simulink model "Lab3"  (Simulink 7.1)
settings: Solver=ode45  SolverMode=SingleTasking  StartTime=0.0  StopTime=10.0  RelTol=1e-3  AbsTol=1e-6
settings Model: Creator=vise  LastModifiedBy=vise  ExtModeTrigMode=oneshot  ExtModeArmWhenConnect=off
settings DataIOCC: LimitDataPoints=off
settings OptimizationCC: BlockReduction=off  BooleanDataType=off
settings DebuggingCC: SaveWithParameterizedLinksMsg=none  SignalResolutionControl=TryResolveAllWithWarning  SolverPrmCheckMsg=none  MultiTaskDSMMsg=warning  MultiTaskCondExecSysMsg=none  StrictBusMsg=None
settings HardwareCC: TargetUnknown=on
settings RTWCC: TemplateMakefile=grt_unix.tmf  IncludeERTFirstTime=on

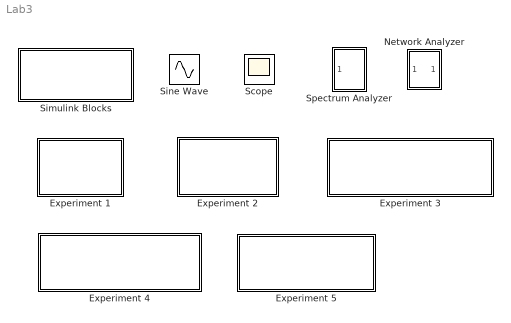
== system Lab3 ==
  Experiment 1 : Subsystem
      settings: OpenFcn=lab3Synth
      mask Type: Waveform Synthesizer
      mask Display: disp('Synthesizer')
  Experiment 2 : Subsystem
      settings: OpenFcn=lab3Mod
      mask Type: Modulator
      mask Display: disp('Modulator')
  Experiment 3 : Subsystem  Orientation=left
      settings: OpenFcn=lab3CTSys1
      mask Type: CT System Analysis/Network Analyzer
      mask Display: disp('CT System Analysis using\n a Network Analyzer')
  Experiment 4 : Subsystem
      settings: OpenFcn=lab3CTSys2
      mask Type: CT System Analysis/Unit Step
      mask Display: disp('CT System Analysis using\n a Unit Step')
  Experiment 5 : Subsystem
      settings: OpenFcn=lab3DTSys
      mask Type: DT System Analysis
      mask Display: disp('DT System Analysis')
  Network Analyzer : Subsystem  Orientation=left  mask(Network Analyzer){@1=256, @2=0.1}
      mask prompts: @1 "Number of sample points:"; @2 "Sampling period (sec):"
      mask init:
      | max_freq=0.9*pi/@2;N=@1;T_s=@2;const=2*pi/(@1*@2);window1=0.5*@1*@2;window2=@1*@2;
      mask Help: Estimates frequency response of system using chirp input. Used for EE438. See Prof. Bouman.
      mask Display: plot(0,0,100,100,[11,93,93,11,11],[90,90,40,40,90],[80,60,40,20],[50,79,50,80])
  Scope : Scope
      settings: TickLabels=on  DataFormat=Array
  Simulink Blocks : Subsystem
      settings: OpenFcn=simulink
      mask Type: Waveform Synthesizer
      mask Display: disp('Full Block Library')
  Sine Wave : Sin  SampleTime=0
  Spectrum Analyzer : Subsystem  mask(Spectrum analyzer.){@1=2048, @2=0.02, @3=10}
      mask prompts: @1 "Number of sample points:"; @2 "Sampling period (sec):"; @3 "Plotting Period (sec):"
      mask init:
      | N=@1; T_s=@2;plot_period=@3;
      mask Help: EE438 Lab utility; See Prof. Bouman.
      mask Display: plot(0,0,100,100,[14,91,91,14,14],[86,86,40,40,86],[85,82,80,79,75,67,63,60,57,53,41,36,33,27,24],[49,50,53,50,49,51,54,66,54,50,50,52,81,51,49])

== system Lab3/Experiment 1 ==

== system Lab3/Experiment 2 ==

== system Lab3/Experiment 3 ==

== system Lab3/Experiment 4 ==

== system Lab3/Experiment 5 ==

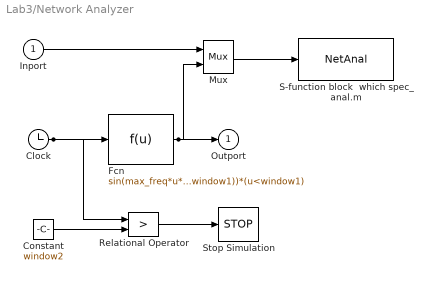
== system Lab3/Network Analyzer ==
  Inport : Inport
  Clock : Clock
      settings: Decimation=10
  Constant : Constant  Value=window2
  Fcn : Fcn  Expr=sin(max_freq*u*u/(2*window1))*(0.54+0.46*cos(pi*u/window1))*(u<window1)
  Mux : Mux  Inputs=2
  Relational Operator : RelationalOperator  Operator=>  InputSameDT=on
  S-function block  which spec_anal.m : S-Function  FunctionName=NetAnal  Parameters=N,T_s  EnableBusSupport=off
  Stop Simulation : Stop
  Outport : Outport  InitialOutput=0
  wires:
  Inport/1 -> Mux/1
  Fcn/1 -> Mux/2, Outport/1
  Mux/1 -> S-function block  which spec_anal.m/1
  Clock/1 -> Fcn/1, Relational Operator/1
  Constant/1 -> Relational Operator/2
  Relational Operator/1 -> Stop Simulation/1

== system Lab3/Simulink Blocks ==

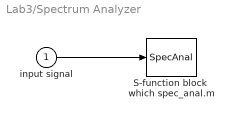
== system Lab3/Spectrum Analyzer ==
  input signal : Inport
  S-function block  which spec_anal.m : S-Function  FunctionName=SpecAnal  Parameters=N,T_s,plot_period  EnableBusSupport=off
  wires:
  input signal/1 -> S-function block  which spec_anal.m/1
